simulink model "model"  (R2016b)
settings: Solver=VariableStepAuto  StartTime=0.0  StopTime=10.0  RelTol=1e-3
settings Model: Creator=庄明宇  LastModifiedBy=庄明宇

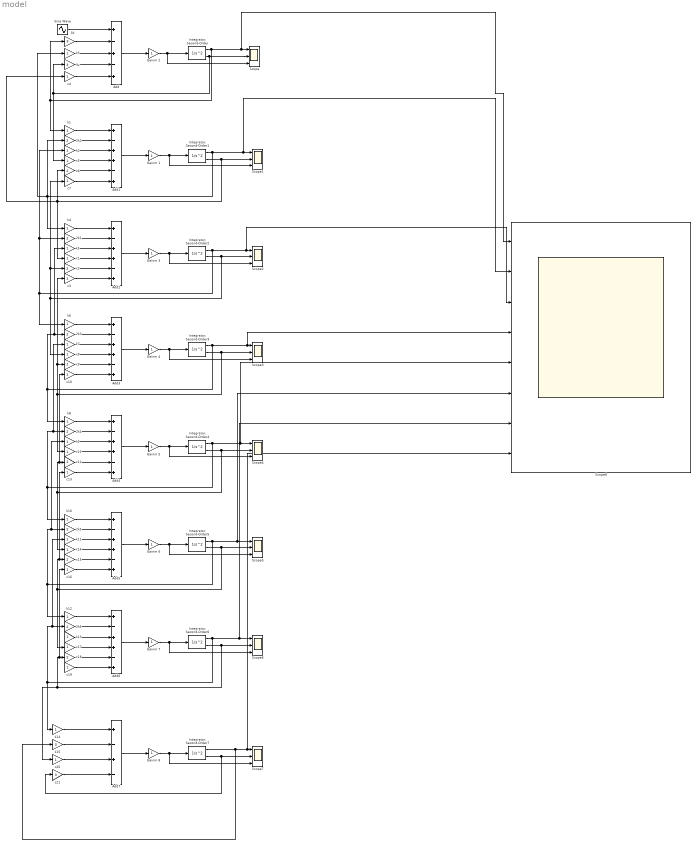
== system model ==
  2k{1..6} (6 alike) : Gain  Gain=2
  3c : Gain  Gain=3
  3k : Gain  Gain=3
  Add : Sum  Inputs=+-+-+
  Add{1..6} (6 alike) : Sum  Inputs=+-++-+
  Add7 : Sum  Inputs=+-+-
  Gainm {1..8} (8 alike) : Gain
  Integrator, Second-Order{,1..7} (8 alike) : SecondOrderIntegrator
  Scope{,1..7} (8 alike) : Scope  NumInputPorts=3
  Scope8 : Scope  NumInputPorts=8
  Sine Wave : Sin  SampleTime=0
  c{1,3..5,7..8,10..11,13..14,16..17,19..20} (14 alike) : Gain
  c{2,6,9,12,15,18} (6 alike) : Gain  Gain=2
  c21 : Gain  Gain=3
  k{1..14} (14 alike) : Gain
  k15 : Gain  Gain=3
  wires:
  Sine Wave/1 -> Add/1
  Gainm 2/1 -> Scope/3, "Integrator, Second-Order"/1
  "Integrator, Second-Order"/1 -> 3k/1, k1/1, Scope8/1, Scope/1
  "Integrator, Second-Order"/2 -> 3c/1, c5/1, Scope/2
  Add/1 -> Gainm 2/1
  3k/1 -> Add/2
  3c/1 -> Add/4
  k1/1 -> Add1/1
  Add1/1 -> Gainm 1/1
  Gainm 1/1 -> Scope1/3, "Integrator, Second-Order1"/1
  "Integrator, Second-Order1"/1 -> k4/1, k3/1, 2k2/1, Scope8/2, Scope1/1
  "Integrator, Second-Order1"/2 -> c1/1, c6/1, c4/1, Scope1/2
  2k2/1 -> Add1/2
  k2/1 -> Add1/3
  k3/1 -> Add/3
  c4/1 -> Add/5
  c5/1 -> Add1/4
  c6/1 -> Add1/5
  c7/1 -> Add1/6
  k4/1 -> Add2/1
  Add2/1 -> Gainm 3/1
  Gainm 3/1 -> Scope2/3, "Integrator, Second-Order2"/1
  "Integrator, Second-Order2"/1 -> k6/1, 2k1/1, k2/1, Scope8/3, Scope2/1
  "Integrator, Second-Order2"/2 -> c8/1, c2/1, c7/1, Scope2/2
  2k1/1 -> Add2/2
  k5/1 -> Add2/3
  c1/1 -> Add2/4
  c2/1 -> Add2/5
  c3/1 -> Add2/6
  k6/1 -> Add3/1
  Add3/1 -> Gainm 4/1
  Gainm 4/1 -> Scope3/3, "Integrator, Second-Order3"/1
  "Integrator, Second-Order3"/1 -> k8/1, k5/1, 2k3/1, Scope8/4, Scope3/1
  "Integrator, Second-Order3"/2 -> c11/1, c9/1, c3/1, Scope3/2
  2k3/1 -> Add3/2
  k7/1 -> Add3/3
  c8/1 -> Add3/4
  c9/1 -> Add3/5
  c10/1 -> Add3/6
  k8/1 -> Add4/1
  Add4/1 -> Gainm 5/1
  Gainm 5/1 -> Scope4/3, "Integrator, Second-Order4"/1
  "Integrator, Second-Order4"/1 -> k10/1, k7/1, 2k4/1, Scope8/5, Scope4/1
  "Integrator, Second-Order4"/2 -> c14/1, c10/1, c12/1, Scope4/2
  2k4/1 -> Add4/2
  k9/1 -> Add4/3
  c11/1 -> Add4/4
  c12/1 -> Add4/5
  c13/1 -> Add4/6
  k10/1 -> Add5/1
  Add5/1 -> Gainm 6/1
  Gainm 6/1 -> Scope5/3, "Integrator, Second-Order5"/1
  "Integrator, Second-Order5"/1 -> k12/1, k9/1, 2k5/1, Scope8/6, Scope5/1
  "Integrator, Second-Order5"/2 -> c17/1, c13/1, c15/1, Scope5/2
  2k5/1 -> Add5/2
  k11/1 -> Add5/3
  c14/1 -> Add5/4
  c15/1 -> Add5/5
  c16/1 -> Add5/6
  k12/1 -> Add6/1
  Add6/1 -> Gainm 7/1
  Gainm 7/1 -> Scope6/3, "Integrator, Second-Order6"/1
  "Integrator, Second-Order6"/1 -> k11/1, 2k6/1, k14/1, Scope6/1, Scope8/7
  "Integrator, Second-Order6"/2 -> c20/1, c16/1, c18/1, Scope6/2
  2k6/1 -> Add6/2
  k13/1 -> Add6/3
  c17/1 -> Add6/4
  c18/1 -> Add6/5
  c19/1 -> Add6/6
  Add7/1 -> Gainm 8/1
  Gainm 8/1 -> Scope7/3, "Integrator, Second-Order7"/1
  "Integrator, Second-Order7"/1 -> k15/1, Scope8/8, Scope7/1
  "Integrator, Second-Order7"/2 -> c21/1, Scope7/2
  c20/1 -> Add7/3
  c21/1 -> Add7/4
  k14/1 -> Add7/1
  k15/1 -> Add7/2
